simulink model "Inverted_Pendulum_5_edition"  (R2022a)
settings: Solver=VariableStepAuto  StartTime=0.0  StopTime=10.0  RelTol=1e-3
settings Model: Creator=Electronica Care  LastModifiedBy=Electronica Care

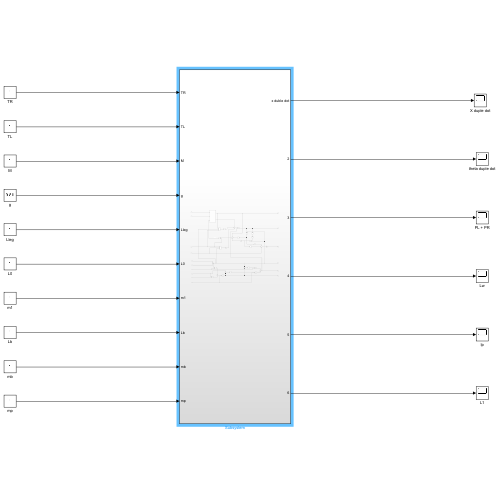
[thumbnail: Simulink's stored preview of the top-level diagram]
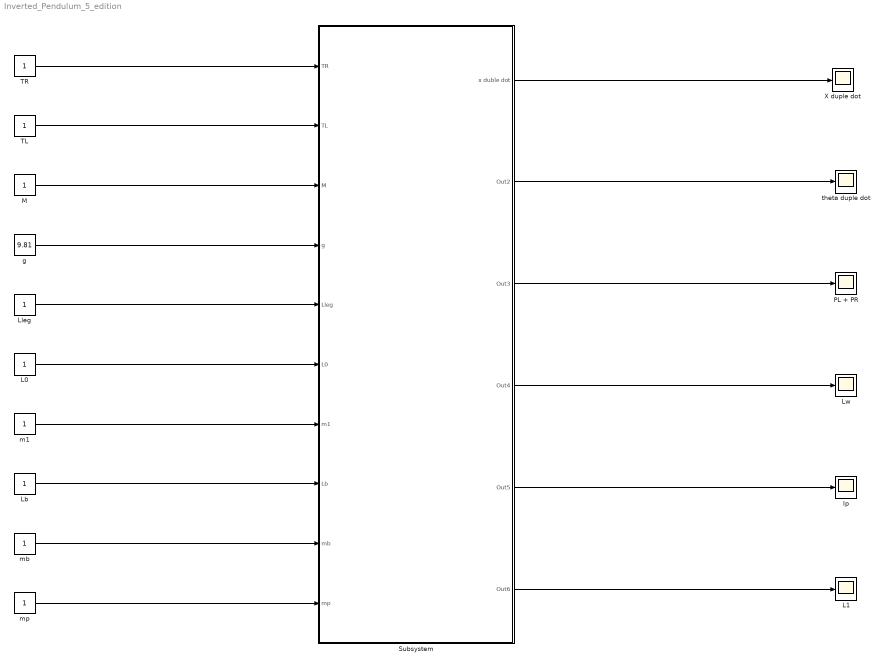
== system Inverted_Pendulum_5_edition ==
  Ip : Scope
  L0 : Constant
  L1 : Scope
  Lb : Constant
  Lleg : Constant
  Lw : Scope
  M : Constant
  PL + PR : Scope
  Subsystem : Subsystem
  TL : Constant
  TR : Constant
  X duple dot : Scope
  g : Constant  Value=9.81
  m1 : Constant
  mb : Constant
  mp : Constant
  theta duple dot : Scope
  wires:
  TR/1 -> Subsystem/1(TR)
  TL/1 -> Subsystem/2(TL)
  M/1 -> Subsystem/3(M)
  g/1 -> Subsystem/4(g)
  Lleg/1 -> Subsystem/5(Lleg)
  L0/1 -> Subsystem/6(L0)
  m1/1 -> Subsystem/7(m1)
  Lb/1 -> Subsystem/8(Lb)
  mb/1 -> Subsystem/9(mb)
  mp/1 -> Subsystem/10(mp)
  Subsystem/1(x duble dot) -> X duple dot/1
  Subsystem/2(Out2) -> theta duple dot/1
  Subsystem/3(Out3) -> PL + PR/1
  Subsystem/4(Out4) -> Lw/1
  Subsystem/5(Out5) -> Ip/1
  Subsystem/6(Out6) -> L1/1

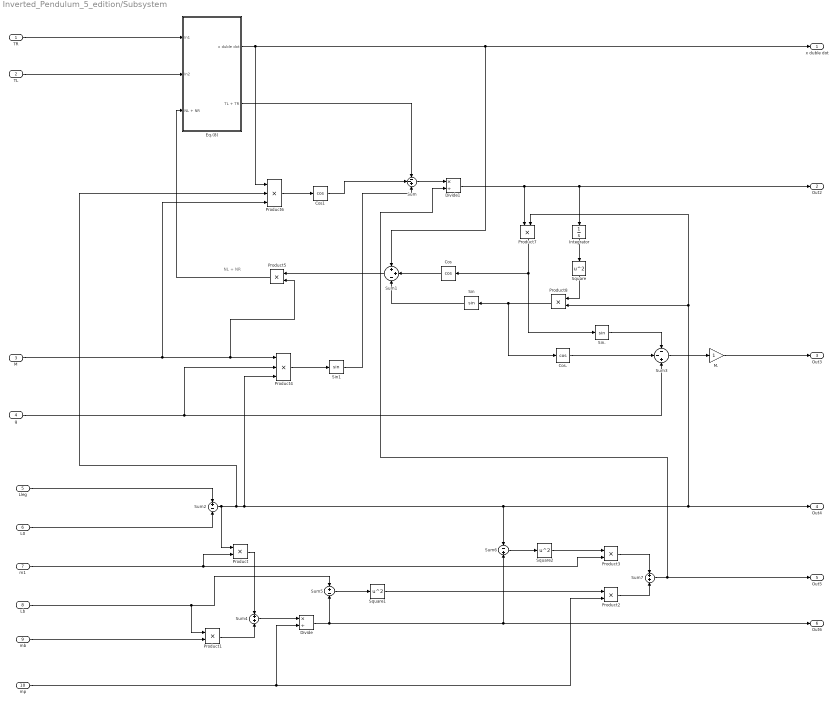
== system Inverted_Pendulum_5_edition/Subsystem ==
  note: NL + NR
  TR : Inport
  TL : Inport  Port=2
  M : Inport  Port=3
  g : Inport  Port=4
  Lleg : Inport  Port=5
  L0 : Inport  Port=6
  m1 : Inport  Port=7
  Lb : Inport  Port=8
  mb : Inport  Port=9
  mp : Inport  Port=10
  Cos : Trigonometry  Operator=cos
  Cos. : Trigonometry  Operator=cos
  Cos1 : Trigonometry  Operator=cos
  Divide : Product  Inputs=*/
  Divide1 : Product  Inputs=*/
  Eq.(8) : Subsystem
  Integrator : Integrator
  M. : Gain
  Product{,1..3,5,7..8} (7 alike) : Product
  Product4 : Product  Inputs=3
  Product6 : Product  Inputs=3
  Sin : Trigonometry
  Sin. : Trigonometry
  Sin1 : Trigonometry
  Square : Math  Operator=square
  Square1 : Math  Operator=square
  Square2 : Math  Operator=square
  Sum : Sum  Inputs=--+
  Sum1 : Sum  Inputs=++-
  Sum2 : Sum  Inputs=+-
  Sum3 : Sum  Inputs=--+
  Sum4 : Sum
  Sum5 : Sum  Inputs=+-
  Sum6 : Sum  Inputs=-+
  Sum7 : Sum
  x duble dot : Outport
  Out2 : Outport  Port=2
  Out3 : Outport  Port=3
  Out4 : Outport  Port=4
  Out5 : Outport  Port=5
  Out6 : Outport  Port=6
  wires:
  Sum2/1 -> Product6/2, Sum6/1, Out4/1, Product7/2, Product8/2, Product4/3, Product/1
  Eq.(8)/2(TL + TR) -> Sum/1
  Product3/1 -> Sum7/1
  Square2/1 -> Product3/1
  Eq.(8)/1(x duble dot) -> x duble dot/1, Sum1/1, Product6/1
  M./1 -> Out3/1
  Sin./1 -> Sum3/1
  Sin/1 -> Sum1/3
  g/1 -> Sum3/3, Product4/2
  m1/1 -> Product3/2, Product/2
  Integrator/1 -> Square/1
  Sum/1 -> Divide1/1
  Cos1/1 -> Sum/2
  Product8/1 -> Cos./1, Sin/1
  Cos./1 -> Sum3/2
  Sum5/1 -> Square1/1
  Sum3/1 -> M./1
  mb/1 -> Product1/2
  Product4/1 -> Sin1/1
  Divide1/1 -> Product7/1, Out2/1, Integrator/1
  M/1 -> Product4/1, Product5/2, Product6/3
  Square/1 -> Product8/1
  Divide/1 -> Sum5/2, Out6/1, Sum6/2
  Product7/1 -> Cos/1, Sin./1
  Sum7/1 -> Out5/1, Divide1/2
  Product2/1 -> Sum7/2
  Product6/1 -> Cos1/1
  TL/1 -> Eq.(8)/2(In2)
  Cos/1 -> Sum1/2
  Product5/1 -> Eq.(8)/3(NL + NR)
  Sum1/1 -> Product5/1
  Product/1 -> Sum4/1
  Product1/1 -> Sum4/2
  Square1/1 -> Product2/1
  Sum6/1 -> Square2/1
  mp/1 -> Product2/2, Divide/2
  Sum4/1 -> Divide/1
  Sin1/1 -> Sum/3
  Lb/1 -> Sum5/1, Product1/1
  Lleg/1 -> Sum2/1
  TR/1 -> Eq.(8)/1(In1)
  L0/1 -> Sum2/2

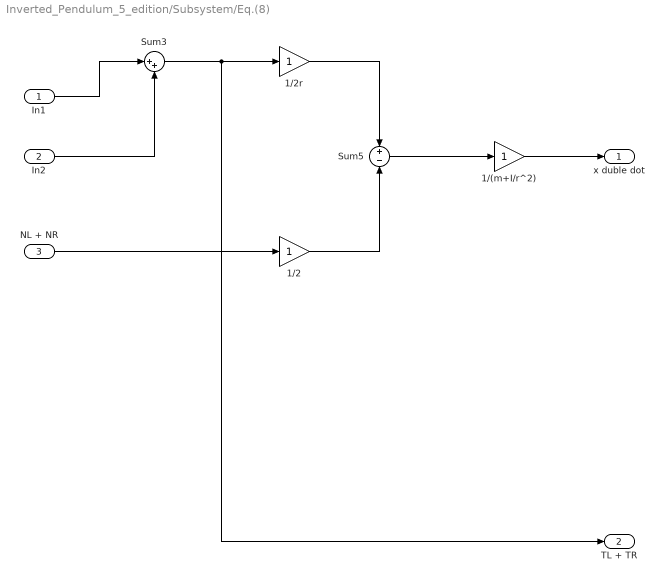
== system Inverted_Pendulum_5_edition/Subsystem/Eq.(8) ==
  In1 : Inport
  In2 : Inport  Port=2
  NL + NR : Inport  Port=3
  1/(m+I/r^2) : Gain
  1/2 : Gain
  1/2r : Gain
  Sum3 : Sum  Inputs=|++
  Sum5 : Sum  Inputs=+-
  x duble dot : Outport
  TL + TR : Outport  Port=2
  wires:
  In1/1 -> Sum3/1
  In2/1 -> Sum3/2
  1/2/1 -> Sum5/2
  1/2r/1 -> Sum5/1
  NL + NR/1 -> 1/2/1
  Sum3/1 -> TL + TR/1, 1/2r/1
  Sum5/1 -> 1/(m+I/r^2)/1
  1/(m+I/r^2)/1 -> x duble dot/1
